simulink model "task_2_sim"  (R2023a)
settings: Solver=VariableStepAuto  StartTime=0.0  StopTime=5  MaxStep=1e-5  RelTol=1e-5
undefined symbols (not defined in the file): A, B, Cz, Dz, G, K1, K2, w_g0, x0
settings Model: Creator=user  LastModifiedBy=user

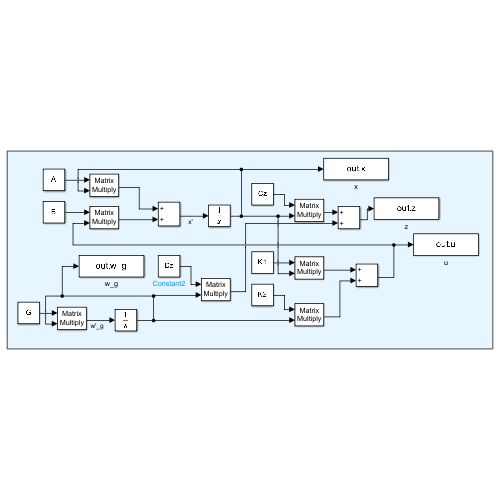
[thumbnail: Simulink's stored preview of the top-level diagram]
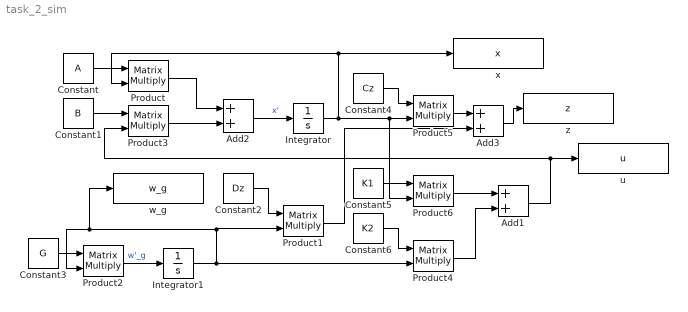
== system task_2_sim ==
  Add1 : Sum
  Add2 : Sum
  Add3 : Sum
  Constant : Constant  Value=A
  Constant1 : Constant  Value=B
  Constant2 : Constant  Value=Dz  VectorParams1D=off
  Constant3 : Constant  Value=G
  Constant4 : Constant  Value=Cz  VectorParams1D=off
  Constant5 : Constant  Value=K1  VectorParams1D=off
  Constant6 : Constant  Value=K2  VectorParams1D=off
  Integrator : Integrator  InitialCondition=x0
  Integrator1 : Integrator  InitialCondition=w_g0
  Product{,1..6} (7 alike) : Product  Multiplication=Matrix(*)
  u : ToWorkspace  VariableName=u  SaveFormat=Timeseries  SampleTime=-1
  w_g : ToWorkspace  VariableName=w_g  SaveFormat=Timeseries  SampleTime=-1
  x : ToWorkspace  VariableName=x  SaveFormat=Timeseries  SampleTime=-1
  z : ToWorkspace  VariableName=z  SaveFormat=Timeseries  SampleTime=-1
  wires:
  Constant/1 -> Product/1
  Constant1/1 -> Product3/1
  Product6/1 -> Add1/1
  Product2/1 -> Integrator1/1  "w'_g"
  Integrator1/1 -> Product2/2, w_g/1, Product1/2, Product4/2
  Constant3/1 -> Product2/1
  Integrator/1 -> Product5/2, Product6/2, x/1, Product/2
  Product3/1 -> Add2/2
  Constant4/1 -> Product5/1
  Product/1 -> Add2/1
  Constant5/1 -> Product6/1
  Product4/1 -> Add1/2
  Add2/1 -> Integrator/1  "x'"
  Constant6/1 -> Product4/1
  Add1/1 -> Product3/2, u/1
  Constant2/1 -> Product1/1
  Product5/1 -> Add3/1
  Product1/1 -> Add3/2
  Add3/1 -> z/1
